simulink model "golayCorrelator"  (R2014b)
settings: Solver=FixedStepDiscrete  StartTime=0  StopTime=10000  RelTol=1e-3
values from neighbouring files (symbols this model uses):
  cbTol = 5    [golay.m]    (also in rev0BB_setup.m = int16(48-4))
  cef_note = cat(2, Gu_512_note, Gv_512_note, Gv_128_note)    [golay.m]    (also in rev0BB_setup.m = int16(cef_note))
  D_128 = [ 1,  8,  2,  4, 16, 32, 64]    [golay.m]    (also in rev0BB_setup.m)
  tol = 15    [golay.m]    (also in rev0BB_setup.m = int16(15+expectedPer*4))
  W_128 = [-1, -1, -1, -1, +1, -1, -1]    [golay.m]    (also in rev0BB_setup.m)
libraries: golayLib x7, commdigbbndpm3 x2, commchan3 x1, dspmlti4 x1, commrflib2 x1, dspsigops x1
settings Model: Creator=cyarp  LastModifiedBy=cyarp

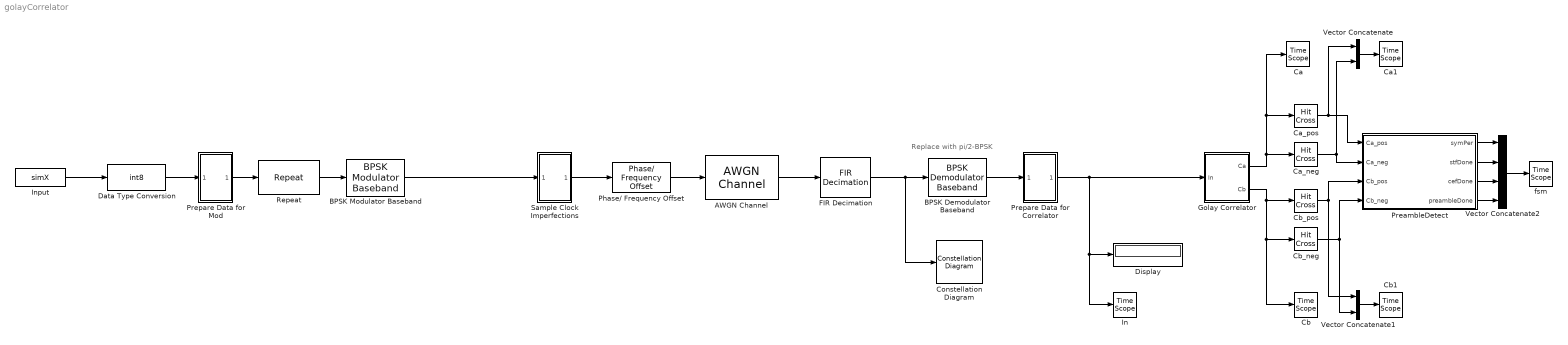
== system golayCorrelator ==
  note: Replace with pi/2-BPSK
  AWGN Channel : commchan3/AWGN Channel  InputProcessing=Columns as channels (frame based)  seed=67  noiseMode="Signal to noise ratio  (Eb/No)"  EbNodB=0  EsNodB=10  SNRdB=10  bitsPerSym=1  Ps=1  Tsym=1  variance=1
  BPSK Demodulator Baseband : commdigbbndpm3/BPSK Demodulator Baseband  Ph=0  DecType=Hard decision  VarSource=Dialog  Variance=1  outDtype=Inherit via internal rule  derotateFactorWordLen=16
  BPSK Modulator Baseband : commdigbbndpm3/BPSK Modulator Baseband  Ph=0  outDtype=double  outWordLen=16  outUDDataType=sfix(16)  outFracLenMode=Best precision  outFracLen=15
  Ca : TimeScope  DefaultConfigurationName=spbscopes.TimeScopeBlockCfg
  Ca1 : TimeScope  DefaultConfigurationName=spbscopes.TimeScopeBlockCfg
  Ca_neg : HitCross  HitCrossingOffset=-50  HitCrossingDirection=falling
  Ca_pos : HitCross  HitCrossingOffset=50  HitCrossingDirection=rising
  Cb : TimeScope  DefaultConfigurationName=spbscopes.TimeScopeBlockCfg
  Cb1 : TimeScope  DefaultConfigurationName=spbscopes.TimeScopeBlockCfg
  Cb_neg : HitCross  HitCrossingOffset=-50  HitCrossingDirection=falling
  Cb_pos : HitCross  HitCrossingOffset=50  HitCrossingDirection=rising
  Constellation Diagram : ConstellationDiagram
  Data Type Conversion : DataTypeConversion  OutDataTypeStr=int8  RndMeth=Nearest
  Display : Display
  FIR Decimation : dspmlti4/FIR Decimation  h=fir1(45, 0.18)  D=4  filtStruct=Direct form  framing=Allow multirate processing  inputOffset=0  outputBufInitCond=0  InputProcessing=Columns as channels (frame based)  firstCoeffDataTypeStr=Inherit: Same word length as input  firstCoeffLastDataTypeStr=Inherit: Same word length as input  firstCoeffMin=[]  firstCoeffMax=[]  outputDataTypeStr=Inherit: Same as accumulator  outputLastDataTypeStr=Inherit: Same as accumulator  outputMin=[]  outputMax=[]  roundingMode=Floor  overflowMode=off  FilterSource=Specify via dialog  FilterObject=Hm_firdecim
      settings: allowOverrides=off
  Golay Correlator : Subsystem
  In : TimeScope  DefaultConfigurationName=spbscopes.TimeScopeBlockCfg
  Input : FromWorkspace  VariableName=simX  SampleTime=1  Interpolate=off  OutputAfterFinalValue=Holding final value
  Phase/ Frequency Offset : commrflib2/Phase// Frequency Offset  phaseOffset=0  freqPort=off  freqOffset=0
  PreambleDetect : Stateflow chart  TreatAsAtomicUnit=on
  Prepare Data for Correlator : Subsystem
  Prepare Data for Mod : Subsystem
  Repeat : dspsigops/Repeat  N=4  InputProcessing=Columns as channels (frame based)  RateOptions=Allow multirate processing  ic=0  mode=Unused parameter value
  Sample Clock Imperfections : Subsystem
  Vector Concatenate : Concatenate  Mode=Multidimensional array  ConcatenateDimension=2
  Vector Concatenate1 : Concatenate  Mode=Multidimensional array  ConcatenateDimension=2
  Vector Concatenate2 : Concatenate  NumInputs=4  Mode=Multidimensional array  ConcatenateDimension=2
  fsm : TimeScope  DefaultConfigurationName=spbscopes.TimeScopeBlockCfg
  wires:
  Phase/ Frequency Offset/1 -> AWGN Channel/1
  Golay Correlator/1(Ca) -> Ca_neg/1, Ca_pos/1, Ca/1
  Golay Correlator/2(Cb) -> Cb_pos/1, Cb_neg/1, Cb/1
  Input/1 -> Data Type Conversion/1
  AWGN Channel/1 -> FIR Decimation/1
  Data Type Conversion/1 -> Prepare Data for Mod/1(In1)
  Prepare Data for Mod/1(Out1) -> Repeat/1
  BPSK Demodulator Baseband/1 -> Prepare Data for Correlator/1(In1)
  Repeat/1 -> BPSK Modulator Baseband/1
  Sample Clock Imperfections/1(Out1) -> Phase/ Frequency Offset/1
  Prepare Data for Correlator/1(Out1) -> In/1, Display/1, Golay Correlator/1(In)
  FIR Decimation/1 -> Constellation Diagram/1, BPSK Demodulator Baseband/1
  Ca_neg/1 -> PreambleDetect/2(Ca_neg), Vector Concatenate/2
  Ca_pos/1 -> PreambleDetect/1(Ca_pos), Vector Concatenate/1
  Vector Concatenate/1 -> Ca1/1
  Cb_pos/1 -> PreambleDetect/3(Cb_pos), Vector Concatenate1/1
  Cb_neg/1 -> Vector Concatenate1/2, PreambleDetect/4(Cb_neg)
  Vector Concatenate1/1 -> Cb1/1
  PreambleDetect/2(stfDone) -> Vector Concatenate2/2
  PreambleDetect/1(symPer) -> Vector Concatenate2/1
  Vector Concatenate2/1 -> fsm/1
  BPSK Modulator Baseband/1 -> Sample Clock Imperfections/1(In1)
  PreambleDetect/3(cefDone) -> Vector Concatenate2/3
  PreambleDetect/4(preambleDone) -> Vector Concatenate2/4

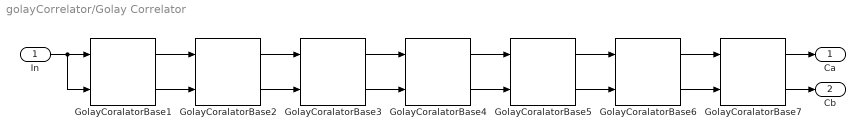
== system golayCorrelator/Golay Correlator ==
  In : Inport
  GolayCoralatorBase1 : golayLib/GolayCoralatorBase  dSub=D_128(1)  wSub=W_128(1)
  GolayCoralatorBase2 : golayLib/GolayCoralatorBase  dSub=D_128(2)  wSub=W_128(2)
  GolayCoralatorBase3 : golayLib/GolayCoralatorBase  dSub=D_128(3)  wSub=W_128(3)
  GolayCoralatorBase4 : golayLib/GolayCoralatorBase  dSub=D_128(4)  wSub=W_128(4)
  GolayCoralatorBase5 : golayLib/GolayCoralatorBase  dSub=D_128(5)  wSub=W_128(5)
  GolayCoralatorBase6 : golayLib/GolayCoralatorBase  dSub=D_128(6)  wSub=W_128(6)
  GolayCoralatorBase7 : golayLib/GolayCoralatorBase  dSub=D_128(7)  wSub=W_128(7)
  Ca : Outport
  Cb : Outport  Port=2
  wires:
  GolayCoralatorBase1/1 -> GolayCoralatorBase2/1
  GolayCoralatorBase1/2 -> GolayCoralatorBase2/2
  GolayCoralatorBase2/1 -> GolayCoralatorBase3/1
  GolayCoralatorBase2/2 -> GolayCoralatorBase3/2
  GolayCoralatorBase5/1 -> GolayCoralatorBase6/1
  GolayCoralatorBase3/1 -> GolayCoralatorBase4/1
  GolayCoralatorBase3/2 -> GolayCoralatorBase4/2
  GolayCoralatorBase4/1 -> GolayCoralatorBase5/1
  GolayCoralatorBase4/2 -> GolayCoralatorBase5/2
  GolayCoralatorBase5/2 -> GolayCoralatorBase6/2
  GolayCoralatorBase6/2 -> GolayCoralatorBase7/2
  GolayCoralatorBase6/1 -> GolayCoralatorBase7/1
  GolayCoralatorBase7/2 -> Cb/1
  GolayCoralatorBase7/1 -> Ca/1
  In/1 -> GolayCoralatorBase1/2, GolayCoralatorBase1/1

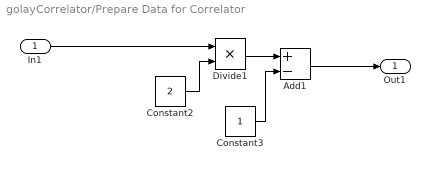
== system golayCorrelator/Prepare Data for Correlator ==
  In1 : Inport
  Add1 : Sum  Inputs=+-
  Constant2 : Constant  Value=2
  Constant3 : Constant
  Divide1 : Product  Inputs=**
  Out1 : Outport
  wires:
  Constant2/1 -> Divide1/2
  Constant3/1 -> Add1/2
  In1/1 -> Divide1/1
  Divide1/1 -> Add1/1
  Add1/1 -> Out1/1

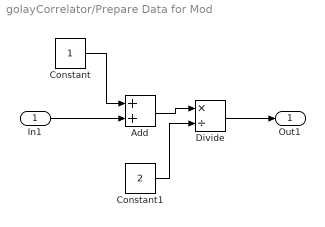
== system golayCorrelator/Prepare Data for Mod ==
  In1 : Inport
  Add : Sum
  Constant : Constant
  Constant1 : Constant  Value=2
  Divide : Product  Inputs=*/
  Out1 : Outport
  wires:
  In1/1 -> Add/2
  Constant/1 -> Add/1
  Add/1 -> Divide/1
  Constant1/1 -> Divide/2
  Divide/1 -> Out1/1

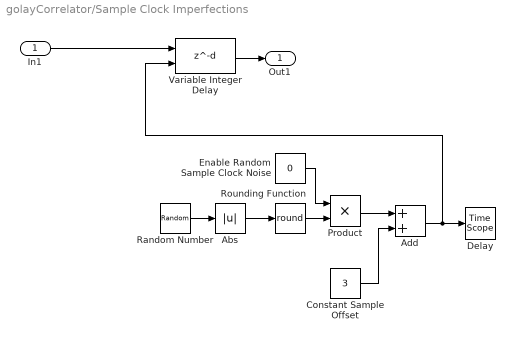
== system golayCorrelator/Sample Clock Imperfections ==
  In1 : Inport
  Abs : Abs
  Add : Sum
  Constant Sample Offset : Constant  Value=3
  Delay : TimeScope  DefaultConfigurationName=spbscopes.TimeScopeBlockCfg
  Enable Random Sample Clock Noise : Constant  Value=0
  Product : Product
  Random Number : RandomNumber  Mean=1  SampleTime=0.25
  Rounding Function : Rounding  Operator=round
  Variable Integer Delay : Delay  DelayLengthSource=Input port
      settings: InputPortMap=u0,p1
  Out1 : Outport
  wires:
  Abs/1 -> Rounding Function/1
  Random Number/1 -> Abs/1
  Add/1 -> Delay/1, Variable Integer Delay/2
  Enable Random Sample Clock Noise/1 -> Product/1
  Constant Sample Offset/1 -> Add/2
  Rounding Function/1 -> Product/2
  Product/1 -> Add/1
  In1/1 -> Variable Integer Delay/1
  Variable Integer Delay/1 -> Out1/1

== stateflow chart golayCorrelator/PreambleDetect ==
  state Preamble
    state STF
      state STF_Neg
        entry:
        symPer = (symPer + counter)/2;
        cbCount = cbCount + 1;
        counter = 1;
        during:
        counter = counter +1;
      state STF_Initial
        entry:
        symPer = (symPer + counter)/2;
        cbCount = cbCount + 1;
        counter = 1;
        during:
        counter = counter +1;
      STF_Initial -> STF_Initial [order 3] : [Cb_pos == 1]
      STF_Initial -> STF_Neg [order 5] : [Cb_neg == 1]
    state CEF
      note: Need actual logic for CEF, right now only checks for correct sequence
      state STF_Done
        entry:
        stfDone = 1;
        symPer = (symPer + counter)/2;
        cbCount = cbCount + 1;
        counter = 1;
        during:
        counter = counter +1;
      state CEF_Checking
        entry:
        symPer = (symPer + counter)/2;
        cefCount = cefCount + 1;
        counter = 1;
        during:
        counter = counter +1;
      STF_Done -> CEF_Checking [order 3] : [Cb_neg == 1]/{
          | cefCount = 1;
          | }
    CEF_Checking -> CEF_Checking [order 2] : [cefSeqCheck(Ca_pos,Ca_neg,Cb_pos, Cb_neg, cefCount) == 1 && cefCount < length(cef_note)]
    STF_Neg -> STF_Done [order 3] : [Ca_neg == 1]
  state Waiting
    entry:
    stfDone = 0;
    cefDone = 0;
    preambleDone = 0;
  state Done
    entry:
    cefDone = 1;
    preambleDone = 1;
  Done -> Waiting
  CEF_Checking -> Waiting [order 4] : [cefSeqCheck(Ca_pos,Ca_neg,Cb_pos, Cb_neg, cefCount) == 1 && counter <(128-tol)]
  STF_Done -> Waiting [order 2] : [Cb_neg == 1 && counter <(128-tol)]
  STF_Neg -> Waiting [order 2] : [Ca_neg == 1 && counter <(128-tol)]
  STF_Initial -> Waiting [order 1] : [Cb_pos == 1 && counter <(128-tol)]
  STF_Neg -> Waiting [order 1] : [Cb_neg == 1 || Ca_pos == 1 || Cb_pos == 1  || counter >(128+tol)]
  (default) -> Waiting
  Waiting -> STF_Initial : [Cb_pos == 1]/
      | {
      | cbCount = 0;
      | counter = 128;
      | symPer = 128;
      | }
  CEF_Checking -> Waiting [order 1] : [cefSeqCheck(Ca_pos,Ca_neg,Cb_pos, Cb_neg, cefCount) == 0 || counter >(128+tol) || cefCount > length(cef_note)]
  STF_Done -> Waiting [order 1] : [Ca_pos == 1 || Ca_neg == 1 || Cb_pos == 1 || counter >(128+tol)]
  STF_Initial -> Waiting [order 4] : [Ca_pos ==  1 || Ca_neg == 1 || counter >(128+tol) || cbCount > 48 + cbTol]
  STF_Initial -> Waiting [order 2] : [Cb_neg && (cbCount < 48 - cbTol)]
  CEF_Checking -> Done [order 3] : [cefSeqCheck(Ca_pos,Ca_neg,Cb_pos, Cb_neg, cefCount) == 1 && cefCount == length(cef_note)]
  data: Ca_p function_input; Ca_n function_input; Cb_p function_input; Cb_n function_input; cnt function_input; ok function_output; Ca_pos input; Ca_neg input; tol parameter double; Cb_pos input; Cb_neg input; cbTol parameter; symPer output; counter local; cbCount local; stfDone output; cef_note parameter; cefDone output; preambleDone output; cefCount local
  function ok = cefSeqCheck(Ca_p, Ca_n, Cb_p, Cb_n, cnt):
    | function ok = cefSeqCheck(Ca_p, Ca_n, Cb_p, Cb_n, cnt)
    | if(Ca_p == 0 && Ca_n == 0 && Cb_p == 0 && Cb_n == 0)
    |     ok = 2; %% not triggered
    | else
    |     switch(cef_note(cnt))
    |         case 1
    |             if(Ca_p == 1)
    |                 ok = 1;
    |             else
    |                 ok = 0;
    |             end
    |         case 2
    |             if(Cb_p == 1)
    |                 ok = 1;
    |             else
    |                 ok = 0;
    |             end
    |         case -1
    |             if(Ca_n == 1)
    |                 ok = 1;
    |             else
    |                 ok = 0;
    |             end
    |         case -2
    |             if(Cb_n == 1)
    |                 ok = 1;
    |             else
    |                 ok = 0;
    |             end
    |         otherwise
    |             ok = 0;
    |     end
    | end
    | end
